simulink model "MCuC_Harness"  (R2025b)
settings: Solver=ode8  StartTime=0.0  StopTime=10.0  FixedStep=.0001  RelTol=1e-3
undefined symbols (not defined in the file): BMS_Contactor_Command, MC_DC_State, MC_VSM_State, UC_State
libraries: simulink x5
settings Model: DataDictionary=rev3_data.sldd  Creator=matat  LastModifiedBy=matat
settings OptimizationCC: DefaultParameterBehavior=Inlined  EnhancedBackFolding=on  PassReuseOutputArgsThreshold=0.0  OptimizeBlockOrder=speed  DifferentSizesBufferReuse=on  OptimizationCustomize=off
settings DebuggingCC: ParameterTunabilityLossMsg=error
settings SFSimCC: MATLABDynamicMemAlloc=off
settings RTWCC: GPUComputeCapability=3.5
settings CodeAppCC: ForceParamTrailComments=on  OperatorAnnotations=on

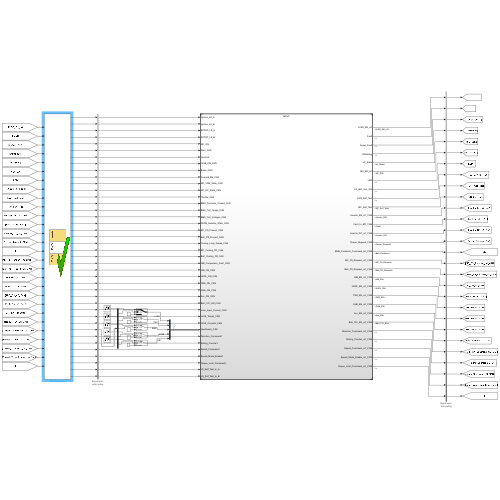
[thumbnail: Simulink's stored preview of the top-level diagram]
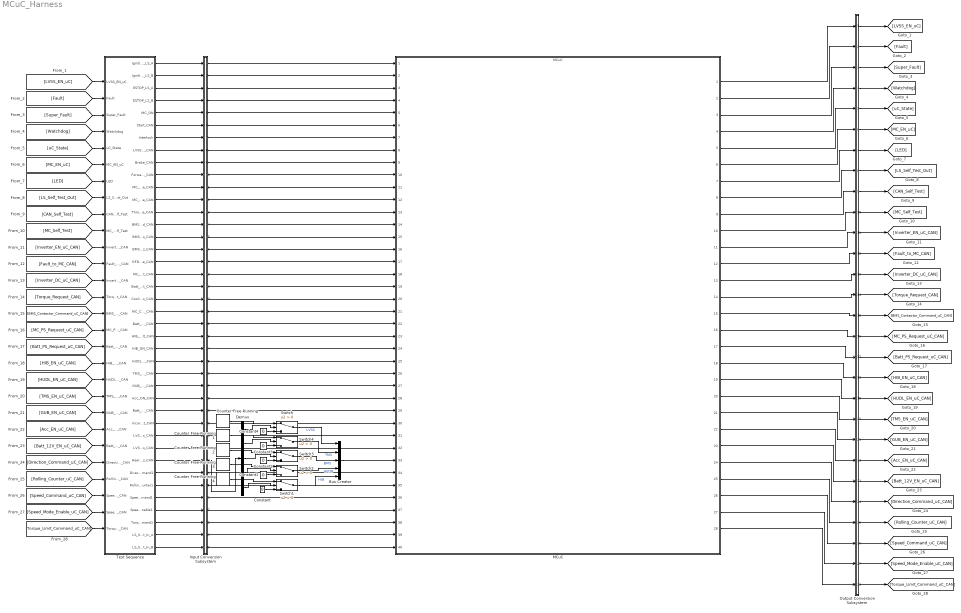
== system MCuC_Harness ==
  Bus Creator : BusCreator  Inputs=5
  Constant{,1..4} (5 alike) : Constant  Value=0
  Counter Free-Running{,1..4} (5 alike) : simulink/Sources/Counter Free-Running  NumBits=32  tsamp=-1
  Demux : Demux  Outputs=5
  Input Conversion Subsystem : Subsystem  Tag=__SLT_ICS__  Description=|
      | Signal spec.
      | and routing
      settings: AttributesFormatString=%<Description>
  MCuC : ModelReference  ModelNameDialog=MCuC  SimulationMode=Normal  ModelReferenceVersion=5.2
  Output Conversion Subsystem : Subsystem  Tag=__SLT_OCS__  Description=|
      | Signal spec.
      | and routing
      settings: AttributesFormatString=%<Description>
  Switch{,1..4} (5 alike) : Switch  Criteria=u2 > Threshold  SaturateOnIntegerOverflow=off  InputSameDT=off
  Test Sequence : Test Sequence  TreatAsAtomicUnit=on
  wires:
  Test Sequence/1(Ignition_LS_A) -> Input Conversion Subsystem/1(Inport_1)
  Test Sequence/2(Ignition_LS_B) -> Input Conversion Subsystem/2(Inport_2)
  Test Sequence/3(ESTOP_LS_A) -> Input Conversion Subsystem/3(Inport_3)
  Test Sequence/4(ESTOP_LS_B) -> Input Conversion Subsystem/4(Inport_4)
  Test Sequence/5(MC_ON) -> Input Conversion Subsystem/5(Inport_5)
  Test Sequence/6(Start_CAN) -> Input Conversion Subsystem/6(Inport_6)
  Test Sequence/7(Interlock) -> Input Conversion Subsystem/7(Inport_7)
  Test Sequence/8(LVSS_ON_CAN) -> Input Conversion Subsystem/8(Inport_8)
  Test Sequence/9(Brake_CAN) -> Input Conversion Subsystem/9(Inport_9)
  Test Sequence/10(Forward_EN_CAN) -> Input Conversion Subsystem/10(Inport_10)
  Test Sequence/11(MC_VSM_State_CAN) -> Input Conversion Subsystem/11(Inport_11)
  Test Sequence/12(MC_DC_State_CAN) -> Input Conversion Subsystem/12(Inport_12)
  Test Sequence/13(Throttle_CAN) -> Input Conversion Subsystem/13(Inport_13)
  Test Sequence/14(BMS_Contactor_Closed_CAN) -> Input Conversion Subsystem/14(Inport_14)
  Test Sequence/15(BMS_Cell_Temps_CAN) -> Input Conversion Subsystem/15(Inport_15)
  Test Sequence/16(BMS_Cell_Voltages_CAN) -> Input Conversion Subsystem/16(Inport_16)
  Test Sequence/17(GFDB_Isolation_State_CAN) -> Input Conversion Subsystem/17(Inport_17)
  Test Sequence/18(MC_PS_Present_CAN) -> Input Conversion Subsystem/18(Inport_18)
  Test Sequence/19(Batt_PS_Present_CAN) -> Input Conversion Subsystem/19(Inport_19)
  Test Sequence/20(Cooling_Loop_Temps_CAN) -> Input Conversion Subsystem/20(Inport_20)
  Test Sequence/21(MC_Cooling_FR_CAN) -> Input Conversion Subsystem/21(Inport_21)
  Test Sequence/22(Batt_Cooling_FR_CAN) -> Input Conversion Subsystem/22(Inport_22)
  Test Sequence/23(HIB_Comparison_Fault_CAN) -> Input Conversion Subsystem/23(Inport_23)
  Test Sequence/24(HIB_ON_CAN) -> Input Conversion Subsystem/24(Inport_24)
  Test Sequence/25(HUDL_ON_CAN) -> Input Conversion Subsystem/25(Inport_25)
  Test Sequence/26(TMS_ON_CAN) -> Input Conversion Subsystem/26(Inport_26)
  Test Sequence/27(GUB_ON_CAN) -> Input Conversion Subsystem/27(Inport_27)
  Test Sequence/28(Acc_ON_CAN) -> Input Conversion Subsystem/28(Inport_28)
  Test Sequence/29(Batt_12V_ON_CAN) -> Input Conversion Subsystem/29(Inport_29)
  Test Sequence/30(Vicor_Input_Current_CAN) -> Input Conversion Subsystem/30(Inport_30)
  Test Sequence/31(LVSS_Temps_CAN) -> Input Conversion Subsystem/31(Inport_31)
  Test Sequence/32(LVSS_Currents_CAN) -> Input Conversion Subsystem/32(Inport_32)
  Test Sequence/34(Direction_Command1) -> Input Conversion Subsystem/34(Inport_34)
  Test Sequence/35(Rolling_Counter1) -> Input Conversion Subsystem/35(Inport_35)
  Test Sequence/36(Speed_Command1) -> Input Conversion Subsystem/36(Inport_36)
  Test Sequence/37(Speed_Mode_Enable1) -> Input Conversion Subsystem/37(Inport_37)
  Test Sequence/38(Torque_Limit_Command1) -> Input Conversion Subsystem/38(Inport_38)
  Test Sequence/39(LS_Self_Test_In_A) -> Input Conversion Subsystem/39(Inport_39)
  Test Sequence/40(LS_Self_Test_In_B) -> Input Conversion Subsystem/40(Inport_40)
  [LVSS_EN_uC] -> Test Sequence/1(LVSS_EN_uC)
  [Fault] -> Test Sequence/2(Fault)
  [Super_Fault] -> Test Sequence/3(Super_Fault)
  [Watchdog] -> Test Sequence/4(Watchdog)
  [uC_State] -> Test Sequence/5(uC_State)
  [MC_EN_uC] -> Test Sequence/6(MC_EN_uC)
  [LED] -> Test Sequence/7(LED)
  [LS_Self_Test_Out] -> Test Sequence/8(LS_Self_Test_Out)
  [CAN_Self_Test] -> Test Sequence/9(CAN_Self_Test)
  [MC_Self_Test] -> Test Sequence/10(MC_Self_Test)
  [Inverter_EN_uC_CAN] -> Test Sequence/11(Inverter_EN_uC_CAN)
  [Fault_to_MC_CAN] -> Test Sequence/12(Fault_to_MC_CAN)
  [Inverter_DC_uC_CAN] -> Test Sequence/13(Inverter_DC_uC_CAN)
  [Torque_Request_CAN] -> Test Sequence/14(Torque_Request_CAN)
  [BMS_Contactor_Command_uC_CAN] -> Test Sequence/15(BMS_Contactor_Command_uC_CAN)
  [MC_PS_Request_uC_CAN] -> Test Sequence/16(MC_PS_Request_uC_CAN)
  [Batt_PS_Request_uC_CAN] -> Test Sequence/17(Batt_PS_Request_uC_CAN)
  [HIB_EN_uC_CAN] -> Test Sequence/18(HIB_EN_uC_CAN)
  [HUDL_EN_uC_CAN] -> Test Sequence/19(HUDL_EN_uC_CAN)
  [TMS_EN_uC_CAN] -> Test Sequence/20(TMS_EN_uC_CAN)
  [GUB_EN_uC_CAN] -> Test Sequence/21(GUB_EN_uC_CAN)
  [Acc_EN_uC_CAN] -> Test Sequence/22(Acc_EN_uC_CAN)
  [Batt_12V_EN_uC_CAN] -> Test Sequence/23(Batt_12V_EN_uC_CAN)
  [Direction_Command_uC_CAN] -> Test Sequence/24(Direction_Command_uC_CAN)
  [Rolling_Counter_uC_CAN] -> Test Sequence/25(Rolling_Counter_uC_CAN)
  [Speed_Command_uC_CAN] -> Test Sequence/26(Speed_Command_uC_CAN)
  [Speed_Mode_Enable_uC_CAN] -> Test Sequence/27(Speed_Mode_Enable_uC_CAN)
  [Torque_Limit_Command_uC_CAN] -> Test Sequence/28(Torque_Limit_Command_uC_CAN)
  Output Conversion Subsystem/1(Outport_1) -> [LVSS_EN_uC]
  Output Conversion Subsystem/2(Outport_2) -> [Fault]
  Output Conversion Subsystem/3(Outport_3) -> [Super_Fault]
  Output Conversion Subsystem/4(Outport_4) -> [Watchdog]
  Output Conversion Subsystem/5(Outport_5) -> [uC_State]
  Output Conversion Subsystem/6(Outport_6) -> [MC_EN_uC]
  Output Conversion Subsystem/7(Outport_7) -> [LED]
  Output Conversion Subsystem/8(Outport_8) -> [LS_Self_Test_Out]
  Output Conversion Subsystem/9(Outport_9) -> [CAN_Self_Test]
  Output Conversion Subsystem/10(Outport_10) -> [MC_Self_Test]
  Output Conversion Subsystem/11(Outport_11) -> [Inverter_EN_uC_CAN]
  Output Conversion Subsystem/12(Outport_12) -> [Fault_to_MC_CAN]
  Output Conversion Subsystem/13(Outport_13) -> [Inverter_DC_uC_CAN]
  Output Conversion Subsystem/14(Outport_14) -> [Torque_Request_CAN]
  Output Conversion Subsystem/15(Outport_15) -> [BMS_Contactor_Command_uC_CAN]
  Output Conversion Subsystem/16(Outport_16) -> [MC_PS_Request_uC_CAN]
  Output Conversion Subsystem/17(Outport_17) -> [Batt_PS_Request_uC_CAN]
  Output Conversion Subsystem/18(Outport_18) -> [HIB_EN_uC_CAN]
  Output Conversion Subsystem/19(Outport_19) -> [HUDL_EN_uC_CAN]
  Output Conversion Subsystem/20(Outport_20) -> [TMS_EN_uC_CAN]
  Output Conversion Subsystem/21(Outport_21) -> [GUB_EN_uC_CAN]
  Output Conversion Subsystem/22(Outport_22) -> [Acc_EN_uC_CAN]
  Output Conversion Subsystem/23(Outport_23) -> [Batt_12V_EN_uC_CAN]
  Output Conversion Subsystem/24(Outport_24) -> [Direction_Command_uC_CAN]
  Output Conversion Subsystem/25(Outport_25) -> [Rolling_Counter_uC_CAN]
  Output Conversion Subsystem/26(Outport_26) -> [Speed_Command_uC_CAN]
  Output Conversion Subsystem/27(Outport_27) -> [Speed_Mode_Enable_uC_CAN]
  Output Conversion Subsystem/28(Outport_28) -> [Torque_Limit_Command_uC_CAN]
  Input Conversion Subsystem/1(Outport_1) -> MCuC/1
  Input Conversion Subsystem/2(Outport_2) -> MCuC/2
  Input Conversion Subsystem/3(Outport_3) -> MCuC/3
  Input Conversion Subsystem/4(Outport_4) -> MCuC/4
  Input Conversion Subsystem/5(Outport_5) -> MCuC/5
  Input Conversion Subsystem/6(Outport_6) -> MCuC/6
  Input Conversion Subsystem/7(Outport_7) -> MCuC/7
  Input Conversion Subsystem/8(Outport_8) -> MCuC/8
  Input Conversion Subsystem/9(Outport_9) -> MCuC/9
  Input Conversion Subsystem/10(Outport_10) -> MCuC/10
  Input Conversion Subsystem/11(Outport_11) -> MCuC/11
  Input Conversion Subsystem/12(Outport_12) -> MCuC/12
  Input Conversion Subsystem/13(Outport_13) -> MCuC/13
  Input Conversion Subsystem/14(Outport_14) -> MCuC/14
  Input Conversion Subsystem/15(Outport_15) -> MCuC/15
  Input Conversion Subsystem/16(Outport_16) -> MCuC/16
  Input Conversion Subsystem/17(Outport_17) -> MCuC/17
  Input Conversion Subsystem/18(Outport_18) -> MCuC/18
  Input Conversion Subsystem/19(Outport_19) -> MCuC/19
  Input Conversion Subsystem/20(Outport_20) -> MCuC/20
  Input Conversion Subsystem/21(Outport_21) -> MCuC/21
  Input Conversion Subsystem/22(Outport_22) -> MCuC/22
  Input Conversion Subsystem/23(Outport_23) -> MCuC/23
  Input Conversion Subsystem/24(Outport_24) -> MCuC/24
  Input Conversion Subsystem/25(Outport_25) -> MCuC/25
  Input Conversion Subsystem/26(Outport_26) -> MCuC/26
  Input Conversion Subsystem/27(Outport_27) -> MCuC/27
  Input Conversion Subsystem/28(Outport_28) -> MCuC/28
  Input Conversion Subsystem/29(Outport_29) -> MCuC/29
  Input Conversion Subsystem/30(Outport_30) -> MCuC/30
  Input Conversion Subsystem/31(Outport_31) -> MCuC/31
  Input Conversion Subsystem/32(Outport_32) -> MCuC/32
  Input Conversion Subsystem/34(Outport_34) -> MCuC/34
  Input Conversion Subsystem/35(Outport_35) -> MCuC/35
  Input Conversion Subsystem/36(Outport_36) -> MCuC/36
  Input Conversion Subsystem/37(Outport_37) -> MCuC/37
  Input Conversion Subsystem/38(Outport_38) -> MCuC/38
  Input Conversion Subsystem/39(Outport_39) -> MCuC/39
  Input Conversion Subsystem/40(Outport_40) -> MCuC/40
  MCuC/1 -> Output Conversion Subsystem/1(Inport_1)
  MCuC/2 -> Output Conversion Subsystem/2(Inport_2)
  MCuC/3 -> Output Conversion Subsystem/3(Inport_3)
  MCuC/4 -> Output Conversion Subsystem/4(Inport_4)
  MCuC/5 -> Output Conversion Subsystem/5(Inport_5)
  MCuC/6 -> Output Conversion Subsystem/6(Inport_6)
  MCuC/7 -> Output Conversion Subsystem/7(Inport_7)
  MCuC/8 -> Output Conversion Subsystem/8(Inport_8)
  MCuC/9 -> Output Conversion Subsystem/9(Inport_9)
  MCuC/10 -> Output Conversion Subsystem/10(Inport_10)
  MCuC/11 -> Output Conversion Subsystem/11(Inport_11)
  MCuC/12 -> Output Conversion Subsystem/12(Inport_12)
  MCuC/13 -> Output Conversion Subsystem/13(Inport_13)
  MCuC/14 -> Output Conversion Subsystem/14(Inport_14)
  MCuC/15 -> Output Conversion Subsystem/15(Inport_15)
  MCuC/16 -> Output Conversion Subsystem/16(Inport_16)
  MCuC/17 -> Output Conversion Subsystem/17(Inport_17)
  MCuC/18 -> Output Conversion Subsystem/18(Inport_18)
  MCuC/19 -> Output Conversion Subsystem/19(Inport_19)
  MCuC/20 -> Output Conversion Subsystem/20(Inport_20)
  MCuC/21 -> Output Conversion Subsystem/21(Inport_21)
  MCuC/22 -> Output Conversion Subsystem/22(Inport_22)
  MCuC/23 -> Output Conversion Subsystem/23(Inport_23)
  MCuC/24 -> Output Conversion Subsystem/24(Inport_24)
  MCuC/25 -> Output Conversion Subsystem/25(Inport_25)
  MCuC/26 -> Output Conversion Subsystem/26(Inport_26)
  MCuC/27 -> Output Conversion Subsystem/27(Inport_27)
  MCuC/28 -> Output Conversion Subsystem/28(Inport_28)
  Counter Free-Running/1 -> Switch/1
  Counter Free-Running1/1 -> Switch4/1
  Counter Free-Running2/1 -> Switch3/1
  Counter Free-Running3/1 -> Switch2/1
  Counter Free-Running4/1 -> Switch1/1
  Constant/1 -> Switch1/3
  Constant4/1 -> Switch/3
  Constant3/1 -> Switch4/3
  Constant2/1 -> Switch3/3
  Constant1/1 -> Switch2/3
  Test Sequence/33(Heartbeats_CAN) -> Input Conversion Subsystem/33(Inport_33)
  Input Conversion Subsystem/33(Outport_33) -> Demux/1
  Demux/1 -> Switch/2
  Demux/2 -> Switch4/2
  Demux/3 -> Switch3/2
  Demux/4 -> Switch2/2
  Demux/5 -> Switch1/2
  Switch/1 -> Bus Creator/1  "LVSS"
  Switch4/1 -> Bus Creator/2  "TMS"
  Switch3/1 -> Bus Creator/3  "BMS"
  Switch2/1 -> Bus Creator/4  "GFDB"
  Switch1/1 -> Bus Creator/5  "HIB"
  Bus Creator/1 -> MCuC/33

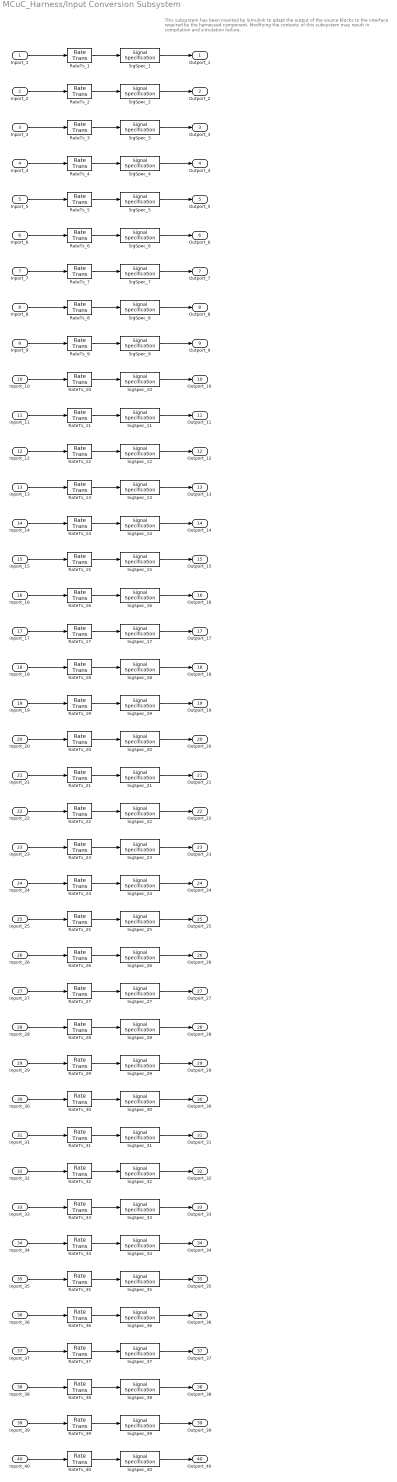
== system MCuC_Harness/Input Conversion Subsystem ==
  note: This subsystem has been inserted by Simulink to adapt the output of the source blocks to the interface required by the harnessed component.
      |  Modifying the contents of this subsystem may result in compilation and simulation failure.
  Inport_1 : Inport
  Inport_2 : Inport  Port=2
  Inport_3 : Inport  Port=3
  Inport_4 : Inport  Port=4
  Inport_5 : Inport  Port=5
  Inport_6 : Inport  Port=6
  Inport_7 : Inport  Port=7
  Inport_8 : Inport  Port=8
  Inport_9 : Inport  Port=9
  Inport_10 : Inport  Port=10
  Inport_11 : Inport  Port=11
  Inport_12 : Inport  Port=12
  Inport_13 : Inport  Port=13
  Inport_14 : Inport  Port=14
  Inport_15 : Inport  Port=15
  Inport_16 : Inport  Port=16
  Inport_17 : Inport  Port=17
  Inport_18 : Inport  Port=18
  Inport_19 : Inport  Port=19
  Inport_20 : Inport  Port=20
  Inport_21 : Inport  Port=21
  Inport_22 : Inport  Port=22
  Inport_23 : Inport  Port=23
  Inport_24 : Inport  Port=24
  Inport_25 : Inport  Port=25
  Inport_26 : Inport  Port=26
  Inport_27 : Inport  Port=27
  Inport_28 : Inport  Port=28
  Inport_29 : Inport  Port=29
  Inport_30 : Inport  Port=30
  Inport_31 : Inport  Port=31
  Inport_32 : Inport  Port=32
  Inport_33 : Inport  Port=33
  Inport_34 : Inport  Port=34
  Inport_35 : Inport  Port=35
  Inport_36 : Inport  Port=36
  Inport_37 : Inport  Port=37
  Inport_38 : Inport  Port=38
  Inport_39 : Inport  Port=39
  Inport_40 : Inport  Port=40
  RateTs_{1..10,13..40} (38 alike) : RateTransition  OutPortSampleTime=0.0001
  RateTs_11 : RateTransition  InitialCondition=MC_VSM_State.Start  OutPortSampleTime=0.0001
  RateTs_12 : RateTransition  InitialCondition=MC_DC_State.Disabled  OutPortSampleTime=0.0001
  SigSpec_{1..10,14,23..29,39..40} (20 alike) : SignalSpecification  OutDataTypeStr=boolean  Dimensions=[1]  SampleTime=0.0001
  SigSpec_11 : SignalSpecification  OutDataTypeStr=Enum: MC_VSM_State  Dimensions=[1]  SampleTime=0.0001
  SigSpec_12 : SignalSpecification  OutDataTypeStr=Enum: MC_DC_State  Dimensions=[1]  SampleTime=0.0001
  SigSpec_{13,21..22,30,34..38} (9 alike) : SignalSpecification  OutDataTypeStr=int16  Dimensions=[1]  SampleTime=0.0001
  SigSpec_15 : SignalSpecification  OutDataTypeStr=int32  Dimensions=[1, 45]  SampleTime=0.0001
  SigSpec_16 : SignalSpecification  OutDataTypeStr=int16  Dimensions=[1, 100]  SampleTime=0.0001
  SigSpec_17 : SignalSpecification  OutDataTypeStr=uint8  Dimensions=[1]  SampleTime=0.0001
  SigSpec_18 : SignalSpecification  OutDataTypeStr=uint8  Dimensions=[1]  SampleTime=0.0001
  SigSpec_19 : SignalSpecification  OutDataTypeStr=uint8  Dimensions=[1]  SampleTime=0.0001
  SigSpec_20 : SignalSpecification  OutDataTypeStr=int32  Dimensions=[1, 5]  SampleTime=0.0001
  SigSpec_31 : SignalSpecification  OutDataTypeStr=int32  Dimensions=[1, 6]  SampleTime=0.0001
  SigSpec_32 : SignalSpecification  OutDataTypeStr=int16  Dimensions=[1, 6]  SampleTime=0.0001
  SigSpec_33 : SignalSpecification  OutDataTypeStr=uint32  Dimensions=[1, 5]  SampleTime=0.0001
  Outport_1 : Outport
  Outport_2 : Outport  Port=2
  Outport_3 : Outport  Port=3
  Outport_4 : Outport  Port=4
  Outport_5 : Outport  Port=5
  Outport_6 : Outport  Port=6
  Outport_7 : Outport  Port=7
  Outport_8 : Outport  Port=8
  Outport_9 : Outport  Port=9
  Outport_10 : Outport  Port=10
  Outport_11 : Outport  Port=11
  Outport_12 : Outport  Port=12
  Outport_13 : Outport  Port=13
  Outport_14 : Outport  Port=14
  Outport_15 : Outport  Port=15
  Outport_16 : Outport  Port=16
  Outport_17 : Outport  Port=17
  Outport_18 : Outport  Port=18
  Outport_19 : Outport  Port=19
  Outport_20 : Outport  Port=20
  Outport_21 : Outport  Port=21
  Outport_22 : Outport  Port=22
  Outport_23 : Outport  Port=23
  Outport_24 : Outport  Port=24
  Outport_25 : Outport  Port=25
  Outport_26 : Outport  Port=26
  Outport_27 : Outport  Port=27
  Outport_28 : Outport  Port=28
  Outport_29 : Outport  Port=29
  Outport_30 : Outport  Port=30
  Outport_31 : Outport  Port=31
  Outport_32 : Outport  Port=32
  Outport_33 : Outport  Port=33
  Outport_34 : Outport  Port=34
  Outport_35 : Outport  Port=35
  Outport_36 : Outport  Port=36
  Outport_37 : Outport  Port=37
  Outport_38 : Outport  Port=38
  Outport_39 : Outport  Port=39
  Outport_40 : Outport  Port=40
  wires:
  SigSpec_1/1 -> Outport_1/1
  RateTs_1/1 -> SigSpec_1/1
  Inport_1/1 -> RateTs_1/1
  SigSpec_2/1 -> Outport_2/1
  RateTs_2/1 -> SigSpec_2/1
  Inport_2/1 -> RateTs_2/1
  SigSpec_3/1 -> Outport_3/1
  RateTs_3/1 -> SigSpec_3/1
  Inport_3/1 -> RateTs_3/1
  SigSpec_4/1 -> Outport_4/1
  RateTs_4/1 -> SigSpec_4/1
  Inport_4/1 -> RateTs_4/1
  SigSpec_5/1 -> Outport_5/1
  RateTs_5/1 -> SigSpec_5/1
  Inport_5/1 -> RateTs_5/1
  SigSpec_6/1 -> Outport_6/1
  RateTs_6/1 -> SigSpec_6/1
  Inport_6/1 -> RateTs_6/1
  SigSpec_7/1 -> Outport_7/1
  RateTs_7/1 -> SigSpec_7/1
  Inport_7/1 -> RateTs_7/1
  SigSpec_8/1 -> Outport_8/1
  RateTs_8/1 -> SigSpec_8/1
  Inport_8/1 -> RateTs_8/1
  SigSpec_9/1 -> Outport_9/1
  RateTs_9/1 -> SigSpec_9/1
  Inport_9/1 -> RateTs_9/1
  SigSpec_10/1 -> Outport_10/1
  RateTs_10/1 -> SigSpec_10/1
  Inport_10/1 -> RateTs_10/1
  SigSpec_11/1 -> Outport_11/1
  RateTs_11/1 -> SigSpec_11/1
  Inport_11/1 -> RateTs_11/1
  SigSpec_12/1 -> Outport_12/1
  RateTs_12/1 -> SigSpec_12/1
  Inport_12/1 -> RateTs_12/1
  SigSpec_13/1 -> Outport_13/1
  RateTs_13/1 -> SigSpec_13/1
  Inport_13/1 -> RateTs_13/1
  SigSpec_14/1 -> Outport_14/1
  RateTs_14/1 -> SigSpec_14/1
  Inport_14/1 -> RateTs_14/1
  SigSpec_15/1 -> Outport_15/1
  RateTs_15/1 -> SigSpec_15/1
  Inport_15/1 -> RateTs_15/1
  SigSpec_16/1 -> Outport_16/1
  RateTs_16/1 -> SigSpec_16/1
  Inport_16/1 -> RateTs_16/1
  SigSpec_17/1 -> Outport_17/1
  RateTs_17/1 -> SigSpec_17/1
  Inport_17/1 -> RateTs_17/1
  SigSpec_18/1 -> Outport_18/1
  RateTs_18/1 -> SigSpec_18/1
  Inport_18/1 -> RateTs_18/1
  SigSpec_19/1 -> Outport_19/1
  RateTs_19/1 -> SigSpec_19/1
  Inport_19/1 -> RateTs_19/1
  SigSpec_20/1 -> Outport_20/1
  RateTs_20/1 -> SigSpec_20/1
  Inport_20/1 -> RateTs_20/1
  SigSpec_21/1 -> Outport_21/1
  RateTs_21/1 -> SigSpec_21/1
  Inport_21/1 -> RateTs_21/1
  SigSpec_22/1 -> Outport_22/1
  RateTs_22/1 -> SigSpec_22/1
  Inport_22/1 -> RateTs_22/1
  SigSpec_23/1 -> Outport_23/1
  RateTs_23/1 -> SigSpec_23/1
  Inport_23/1 -> RateTs_23/1
  SigSpec_24/1 -> Outport_24/1
  RateTs_24/1 -> SigSpec_24/1
  Inport_24/1 -> RateTs_24/1
  SigSpec_25/1 -> Outport_25/1
  RateTs_25/1 -> SigSpec_25/1
  Inport_25/1 -> RateTs_25/1
  SigSpec_26/1 -> Outport_26/1
  RateTs_26/1 -> SigSpec_26/1
  Inport_26/1 -> RateTs_26/1
  SigSpec_27/1 -> Outport_27/1
  RateTs_27/1 -> SigSpec_27/1
  Inport_27/1 -> RateTs_27/1
  SigSpec_28/1 -> Outport_28/1
  RateTs_28/1 -> SigSpec_28/1
  Inport_28/1 -> RateTs_28/1
  SigSpec_29/1 -> Outport_29/1
  RateTs_29/1 -> SigSpec_29/1
  Inport_29/1 -> RateTs_29/1
  SigSpec_30/1 -> Outport_30/1
  RateTs_30/1 -> SigSpec_30/1
  Inport_30/1 -> RateTs_30/1
  SigSpec_31/1 -> Outport_31/1
  RateTs_31/1 -> SigSpec_31/1
  Inport_31/1 -> RateTs_31/1
  SigSpec_32/1 -> Outport_32/1
  RateTs_32/1 -> SigSpec_32/1
  Inport_32/1 -> RateTs_32/1
  SigSpec_33/1 -> Outport_33/1
  RateTs_33/1 -> SigSpec_33/1
  Inport_33/1 -> RateTs_33/1
  SigSpec_34/1 -> Outport_34/1
  RateTs_34/1 -> SigSpec_34/1
  Inport_34/1 -> RateTs_34/1
  SigSpec_35/1 -> Outport_35/1
  RateTs_35/1 -> SigSpec_35/1
  Inport_35/1 -> RateTs_35/1
  SigSpec_36/1 -> Outport_36/1
  RateTs_36/1 -> SigSpec_36/1
  Inport_36/1 -> RateTs_36/1
  SigSpec_37/1 -> Outport_37/1
  RateTs_37/1 -> SigSpec_37/1
  Inport_37/1 -> RateTs_37/1
  SigSpec_38/1 -> Outport_38/1
  RateTs_38/1 -> SigSpec_38/1
  Inport_38/1 -> RateTs_38/1
  SigSpec_39/1 -> Outport_39/1
  RateTs_39/1 -> SigSpec_39/1
  Inport_39/1 -> RateTs_39/1
  SigSpec_40/1 -> Outport_40/1
  RateTs_40/1 -> SigSpec_40/1
  Inport_40/1 -> RateTs_40/1

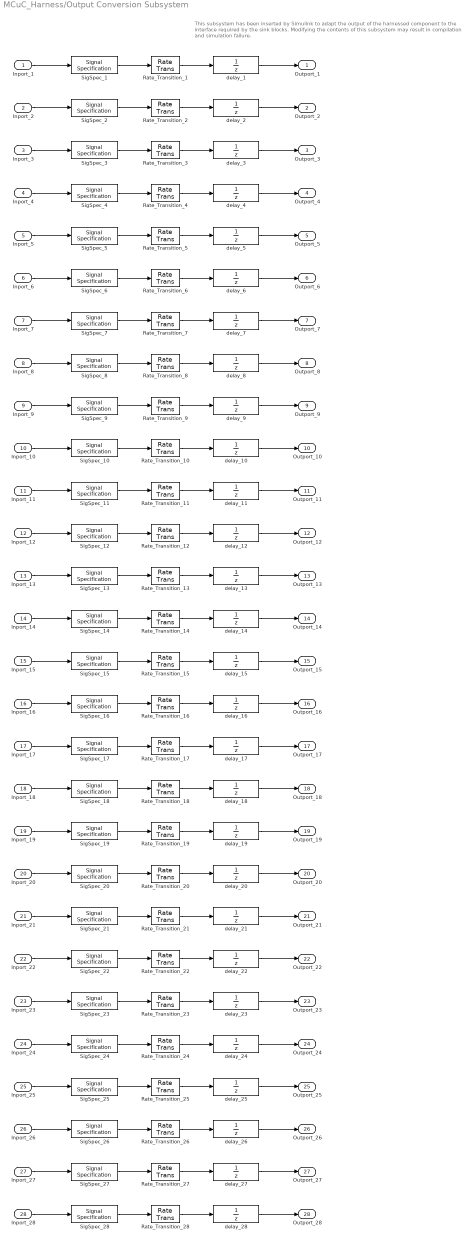
== system MCuC_Harness/Output Conversion Subsystem ==
  note: This subsystem has been inserted by Simulink to adapt the output of the harnessed component to the interface required by the sink blocks.
      |  Modifying the contents of this subsystem may result in compilation and simulation failure.
  Inport_1 : Inport
  Inport_2 : Inport  Port=2
  Inport_3 : Inport  Port=3
  Inport_4 : Inport  Port=4
  Inport_5 : Inport  Port=5
  Inport_6 : Inport  Port=6
  Inport_7 : Inport  Port=7
  Inport_8 : Inport  Port=8
  Inport_9 : Inport  Port=9
  Inport_10 : Inport  Port=10
  Inport_11 : Inport  Port=11
  Inport_12 : Inport  Port=12
  Inport_13 : Inport  Port=13
  Inport_14 : Inport  Port=14
  Inport_15 : Inport  Port=15
  Inport_16 : Inport  Port=16
  Inport_17 : Inport  Port=17
  Inport_18 : Inport  Port=18
  Inport_19 : Inport  Port=19
  Inport_20 : Inport  Port=20
  Inport_21 : Inport  Port=21
  Inport_22 : Inport  Port=22
  Inport_23 : Inport  Port=23
  Inport_24 : Inport  Port=24
  Inport_25 : Inport  Port=25
  Inport_26 : Inport  Port=26
  Inport_27 : Inport  Port=27
  Inport_28 : Inport  Port=28
  Rate_Transition_{1..4,6..14,16..28} (26 alike) : RateTransition  OutPortSampleTimeOpt=Inherit
  Rate_Transition_15 : RateTransition  InitialCondition=BMS_Contactor_Command.Open_Contactor  OutPortSampleTimeOpt=Inherit
  Rate_Transition_5 : RateTransition  InitialCondition=UC_State.Preset  OutPortSampleTimeOpt=Inherit
  SigSpec_{1,4,6,11..13,18..23} (12 alike) : SignalSpecification  OutDataTypeStr=boolean  Dimensions=[1]  SampleTime=0.0001
  SigSpec_{2..3,8..10} (5 alike) : SignalSpecification  OutDataTypeStr=boolean  Dimensions=[1]
  SigSpec_{14,24..28} (6 alike) : SignalSpecification  OutDataTypeStr=int16  Dimensions=[1]  SampleTime=0.0001
  SigSpec_15 : SignalSpecification  OutDataTypeStr=Enum: BMS_Contactor_Command  Dimensions=[1]  SampleTime=0.0001
  SigSpec_16 : SignalSpecification  OutDataTypeStr=uint8  Dimensions=[1]  SampleTime=0.0001
  SigSpec_17 : SignalSpecification  OutDataTypeStr=uint8  Dimensions=[1]  SampleTime=0.0001
  SigSpec_5 : SignalSpecification  OutDataTypeStr=Enum: UC_State  Dimensions=[1]  SampleTime=0.0001
  SigSpec_7 : SignalSpecification  OutDataTypeStr=boolean  Dimensions=[1, 3]  SampleTime=0.0001
  delay_{1..4,6..14,16..28} (26 alike) : UnitDelay  SampleTime=-1
  delay_15 : UnitDelay  InitialCondition=BMS_Contactor_Command.Open_Contactor  SampleTime=-1
  delay_5 : UnitDelay  InitialCondition=UC_State.Preset  SampleTime=-1
  Outport_1 : Outport
  Outport_2 : Outport  Port=2
  Outport_3 : Outport  Port=3
  Outport_4 : Outport  Port=4
  Outport_5 : Outport  Port=5
  Outport_6 : Outport  Port=6
  Outport_7 : Outport  Port=7
  Outport_8 : Outport  Port=8
  Outport_9 : Outport  Port=9
  Outport_10 : Outport  Port=10
  Outport_11 : Outport  Port=11
  Outport_12 : Outport  Port=12
  Outport_13 : Outport  Port=13
  Outport_14 : Outport  Port=14
  Outport_15 : Outport  Port=15
  Outport_16 : Outport  Port=16
  Outport_17 : Outport  Port=17
  Outport_18 : Outport  Port=18
  Outport_19 : Outport  Port=19
  Outport_20 : Outport  Port=20
  Outport_21 : Outport  Port=21
  Outport_22 : Outport  Port=22
  Outport_23 : Outport  Port=23
  Outport_24 : Outport  Port=24
  Outport_25 : Outport  Port=25
  Outport_26 : Outport  Port=26
  Outport_27 : Outport  Port=27
  Outport_28 : Outport  Port=28
  wires:
  Inport_1/1 -> SigSpec_1/1
  SigSpec_1/1 -> Rate_Transition_1/1
  Rate_Transition_1/1 -> delay_1/1
  delay_1/1 -> Outport_1/1
  Inport_2/1 -> SigSpec_2/1
  SigSpec_2/1 -> Rate_Transition_2/1
  Rate_Transition_2/1 -> delay_2/1
  delay_2/1 -> Outport_2/1
  Inport_3/1 -> SigSpec_3/1
  SigSpec_3/1 -> Rate_Transition_3/1
  Rate_Transition_3/1 -> delay_3/1
  delay_3/1 -> Outport_3/1
  Inport_4/1 -> SigSpec_4/1
  SigSpec_4/1 -> Rate_Transition_4/1
  Rate_Transition_4/1 -> delay_4/1
  delay_4/1 -> Outport_4/1
  Inport_5/1 -> SigSpec_5/1
  SigSpec_5/1 -> Rate_Transition_5/1
  Rate_Transition_5/1 -> delay_5/1
  delay_5/1 -> Outport_5/1
  Inport_6/1 -> SigSpec_6/1
  SigSpec_6/1 -> Rate_Transition_6/1
  Rate_Transition_6/1 -> delay_6/1
  delay_6/1 -> Outport_6/1
  Inport_7/1 -> SigSpec_7/1
  SigSpec_7/1 -> Rate_Transition_7/1
  Rate_Transition_7/1 -> delay_7/1
  delay_7/1 -> Outport_7/1
  Inport_8/1 -> SigSpec_8/1
  SigSpec_8/1 -> Rate_Transition_8/1
  Rate_Transition_8/1 -> delay_8/1
  delay_8/1 -> Outport_8/1
  Inport_9/1 -> SigSpec_9/1
  SigSpec_9/1 -> Rate_Transition_9/1
  Rate_Transition_9/1 -> delay_9/1
  delay_9/1 -> Outport_9/1
  Inport_10/1 -> SigSpec_10/1
  SigSpec_10/1 -> Rate_Transition_10/1
  Rate_Transition_10/1 -> delay_10/1
  delay_10/1 -> Outport_10/1
  Inport_11/1 -> SigSpec_11/1
  SigSpec_11/1 -> Rate_Transition_11/1
  Rate_Transition_11/1 -> delay_11/1
  delay_11/1 -> Outport_11/1
  Inport_12/1 -> SigSpec_12/1
  SigSpec_12/1 -> Rate_Transition_12/1
  Rate_Transition_12/1 -> delay_12/1
  delay_12/1 -> Outport_12/1
  Inport_13/1 -> SigSpec_13/1
  SigSpec_13/1 -> Rate_Transition_13/1
  Rate_Transition_13/1 -> delay_13/1
  delay_13/1 -> Outport_13/1
  Inport_14/1 -> SigSpec_14/1
  SigSpec_14/1 -> Rate_Transition_14/1
  Rate_Transition_14/1 -> delay_14/1
  delay_14/1 -> Outport_14/1
  Inport_15/1 -> SigSpec_15/1
  SigSpec_15/1 -> Rate_Transition_15/1
  Rate_Transition_15/1 -> delay_15/1
  delay_15/1 -> Outport_15/1
  Inport_16/1 -> SigSpec_16/1
  SigSpec_16/1 -> Rate_Transition_16/1
  Rate_Transition_16/1 -> delay_16/1
  delay_16/1 -> Outport_16/1
  Inport_17/1 -> SigSpec_17/1
  SigSpec_17/1 -> Rate_Transition_17/1
  Rate_Transition_17/1 -> delay_17/1
  delay_17/1 -> Outport_17/1
  Inport_18/1 -> SigSpec_18/1
  SigSpec_18/1 -> Rate_Transition_18/1
  Rate_Transition_18/1 -> delay_18/1
  delay_18/1 -> Outport_18/1
  Inport_19/1 -> SigSpec_19/1
  SigSpec_19/1 -> Rate_Transition_19/1
  Rate_Transition_19/1 -> delay_19/1
  delay_19/1 -> Outport_19/1
  Inport_20/1 -> SigSpec_20/1
  SigSpec_20/1 -> Rate_Transition_20/1
  Rate_Transition_20/1 -> delay_20/1
  delay_20/1 -> Outport_20/1
  Inport_21/1 -> SigSpec_21/1
  SigSpec_21/1 -> Rate_Transition_21/1
  Rate_Transition_21/1 -> delay_21/1
  delay_21/1 -> Outport_21/1
  Inport_22/1 -> SigSpec_22/1
  SigSpec_22/1 -> Rate_Transition_22/1
  Rate_Transition_22/1 -> delay_22/1
  delay_22/1 -> Outport_22/1
  Inport_23/1 -> SigSpec_23/1
  SigSpec_23/1 -> Rate_Transition_23/1
  Rate_Transition_23/1 -> delay_23/1
  delay_23/1 -> Outport_23/1
  Inport_24/1 -> SigSpec_24/1
  SigSpec_24/1 -> Rate_Transition_24/1
  Rate_Transition_24/1 -> delay_24/1
  delay_24/1 -> Outport_24/1
  Inport_25/1 -> SigSpec_25/1
  SigSpec_25/1 -> Rate_Transition_25/1
  Rate_Transition_25/1 -> delay_25/1
  delay_25/1 -> Outport_25/1
  Inport_26/1 -> SigSpec_26/1
  SigSpec_26/1 -> Rate_Transition_26/1
  Rate_Transition_26/1 -> delay_26/1
  delay_26/1 -> Outport_26/1
  Inport_27/1 -> SigSpec_27/1
  SigSpec_27/1 -> Rate_Transition_27/1
  Rate_Transition_27/1 -> delay_27/1
  delay_27/1 -> Outport_27/1
  Inport_28/1 -> SigSpec_28/1
  SigSpec_28/1 -> Rate_Transition_28/1
  Rate_Transition_28/1 -> delay_28/1
  delay_28/1 -> Outport_28/1

== stateflow chart MCuC_Harness/Test Sequence ==
  state Basic_Operation_Cycle
    state Run
      %% Initialize data outputs.
      Ignition_LS_A = false;
      Ignition_LS_B = false;
      ESTOP_LS_A = false;
      ESTOP_LS_B = false;
      MC_ON = true;
      Start_CAN = false;
      Interlock = true;
      LVSS_ON_CAN = false;
      Brake_CAN = false;
      Forward_EN_CAN = false;
      MC_VSM_State_CAN = MC_VSM_State.Start;
      MC_DC_State_CAN = MC_DC_State.Disabled;
      Throttle_CAN = int16(0);
      BMS_Contactor_Closed_CAN = false;
      BMS_Cell_Temps_CAN = int32(zeros(1, 45));
      BMS_Cell_Voltages_CAN = int16(zeros(1, 100));
      GFDB_Isolation_State_CAN = uint8(0);
      MC_PS_Present_CAN = uint8(0);
      Batt_PS_Present_CAN = uint8(0);
      Cooling_Loop_Temps_CAN = int32(zeros(1, 5));
      MC_Cooling_FR_CAN = int16(0);
      Batt_Cooling_FR_CAN = int16(0);
      HIB_Comparison_Fault_CAN = false;
      HIB_ON_CAN = false;
      HUDL_ON_CAN = false;
      TMS_ON_CAN = false;
      GUB_ON_CAN = false;
      Acc_ON_CAN = false;
      Batt_12V_ON_CAN = false;
      Vicor_Input_Current_CAN = int16(0);
      LVSS_Temps_CAN = int32(zeros(1, 6));
      LVSS_Currents_CAN = int16(zeros(1, 6));
      Heartbeats_CAN = uint32([0, 0, 1, 1, 0]);
      Direction_Command1 = int16(0);
      Rolling_Counter1 = int16(0);
      Speed_Command1 = int16(0);
      Speed_Mode_Enable1 = int16(0);
      Torque_Limit_Command1 = int16(0);
      LS_Self_Test_In_A = false;
      LS_Self_Test_In_B = false;
      verify(BMS_Contactor_Command_uC_CAN == BMS_Contactor_Command.Open_Contactor);
    state Into_Key_Cycle
      BMS_Contactor_Closed_CAN = true;
      MC_ON = false;
    state MC_Off
      verify(LVSS_EN_uC == false);
      verify(Fault == false);
      verify(Super_Fault == false);
      verify(LS_Self_Test_Out == false);
      verify(CAN_Self_Test == false);
      verify(MC_Self_Test == false);
      verify(Inverter_EN_uC_CAN == false);
      verify(Fault_to_MC_CAN == false);
      verify(Inverter_DC_uC_CAN == false);
      verify(Torque_Request_CAN == 0);
      verify(BMS_Contactor_Command_uC_CAN == BMS_Contactor_Command.Close_Contactor);
      verify(MC_PS_Request_uC_CAN == false);
      verify(Batt_PS_Request_uC_CAN == false);
      verify(HIB_EN_uC_CAN == false);
      verify(HUDL_EN_uC_CAN == false);
      verify(TMS_EN_uC_CAN == false);
      verify(GUB_EN_uC_CAN == false);
      verify(Acc_EN_uC_CAN == false);
      verify(Batt_12V_EN_uC_CAN == false);
      verify(Direction_Command_uC_CAN == 0);
      verify(Rolling_Counter_uC_CAN == 0);
      verify(Speed_Command_uC_CAN == 0);
      verify(Speed_Mode_Enable_uC_CAN == 0);
      verify(Torque_Limit_Command_uC_CAN == 0);
      verify(MC_EN_uC == false);
      verify(all(LED ==  [false,true,false]))
      verify(uC_State == UC_State.MC_Off);
      verify(hasChanged(Watchdog) == true)
    state Transition_to_MC_Startup
      Ignition_LS_A = true;
      MC_ON = true;
    state LVSS_MC_Startup
      verify(LVSS_EN_uC == true);
      verify(MC_EN_uC == true);
      verify(uC_State == UC_State.LVSS_MC_Startup);
    state Transition_to_MC_Int
      LVSS_ON_CAN = true;
      Heartbeats_CAN = uint32([1, 0, 1, 1, 0]);
    state MC_Int
      verify(uC_State == UC_State.MC_Init);
      verify(TMS_EN_uC_CAN == true);
      verify(HUDL_EN_uC_CAN == true);
      verify(HIB_EN_uC_CAN == true);
      verify(Batt_12V_EN_uC_CAN == true);
      verify(GUB_EN_uC_CAN == true);
      verify(Acc_EN_uC_CAN == true);
    state Transition_to_Contactor_Closed
      MC_VSM_State_CAN = MC_VSM_State.Ready;
    state Contactor_Closed
      verify(Inverter_EN_uC_CAN == false);
      verify(uC_State == UC_State.Contactor_Closed);
    state Transition_to_MC_Ready
      Heartbeats_CAN = uint32([1, 1, 1, 1, 1]);
      Start_CAN = true;
    state MC_Ready
      verify(Inverter_EN_uC_CAN == false);
      verify(uC_State == UC_State.MC_Ready);
    state Transition_to_MC_Active
      Brake_CAN = true;
      Forward_EN_CAN = true;
      Throttle_CAN = 0;
    state MC_Active
      verify(all(LED ==  [true,false,false]))
      verify(uC_State == UC_State.MC_Active);
    state Transition_to_Contactor_Open
      Ignition_LS_A = false;
      Heartbeats_CAN = uint32([1, 0, 1, 1, 0]);
    state Contactor_Open
      verify(uC_State == UC_State.Contactor_Open);
      verify(TMS_EN_uC_CAN == false);
      verify(HUDL_EN_uC_CAN == false);
      verify(HIB_EN_uC_CAN == false);
      verify(Batt_12V_EN_uC_CAN == false);
      verify(GUB_EN_uC_CAN == false);
      verify(Acc_EN_uC_CAN == false);
      verify(Inverter_DC_uC_CAN == true);
      verify(Inverter_EN_uC_CAN == false);
    state Transition_to_MC_Discharge
      MC_DC_State_CAN = MC_DC_State.Disabled;
      MC_VSM_State_CAN = MC_VSM_State.Shutdown;
    state MC_Discharge
      verify(uC_State == UC_State.MC_Discharging);
    state Transition_to_LVSS_MC_Shutdown
      MC_DC_State_CAN = MC_DC_State.Complete;
      Heartbeats_CAN = uint32([0, 0, 1, 1, 0]);
    state LVSS_MC_Shutdown
      verify(uC_State == UC_State.LVSS_MC_Shutdown);
      verify(MC_EN_uC == false);
      verify(Inverter_DC_uC_CAN == false)
    (default) -> Run
    Run -> Basic_Operation_Cycle.Into_Key_Cycle : [
        | uC_State ~= UC_State.Preset
        | ]
    Basic_Operation_Cycle.Into_Key_Cycle -> MC_Off : [
        | uC_State ~= UC_State.Key_Cycle
        | ]
    MC_Off -> Transition_to_MC_Startup : [
        | after(1, sec)
        | ]
    Transition_to_MC_Startup -> LVSS_MC_Startup : [
        | after(1, sec)
        | ]
    LVSS_MC_Startup -> Transition_to_MC_Int : [
        | after(1, sec)
        | ]
    Transition_to_MC_Int -> MC_Int : [
        | after(1, sec)
        | ]
    MC_Int -> Transition_to_Contactor_Closed : [
        | after(1, sec)
        | ]
    Transition_to_Contactor_Closed -> Contactor_Closed : [
        | after(1, sec)
        | ]
    Contactor_Closed -> Transition_to_MC_Ready : [
        | after(1, sec)
        | ]
    Transition_to_MC_Ready -> MC_Ready : [
        | after(1, sec)
        | ]
    MC_Ready -> Transition_to_MC_Active : [
        | after(1, sec)
        | ]
    Transition_to_MC_Active -> MC_Active : [
        | after(1, sec)
        | ]
    MC_Active -> Transition_to_Contactor_Open : [
        | after(1, sec)
        | ]
    Transition_to_Contactor_Open -> Contactor_Open : [
        | after(1, sec)
        | ]
    Contactor_Open -> Transition_to_MC_Discharge : [
        | after(1, sec)
        | ]
    Transition_to_MC_Discharge -> MC_Discharge : [
        | after(1, sec)
        | ]
    MC_Discharge -> Transition_to_LVSS_MC_Shutdown : [
        | after(1, sec)
        | ]
    Transition_to_LVSS_MC_Shutdown -> LVSS_MC_Shutdown : [
        | after(1, sec)
        | ]
  state Heartbeat_Fault
    state Initialize
      Ignition_LS_A = false;
      Ignition_LS_B = false;
      ESTOP_LS_A = false;
      ESTOP_LS_B = false;
      MC_ON = true;
      Start_CAN = false;
      Interlock = true;
      LVSS_ON_CAN = false;
      Brake_CAN = false;
      Forward_EN_CAN = false;
      MC_VSM_State_CAN = MC_VSM_State.Start;
      MC_DC_State_CAN = MC_DC_State.Disabled;
      Throttle_CAN = int16(0);
      BMS_Contactor_Closed_CAN = false;
      BMS_Cell_Temps_CAN = int32(zeros(1, 45));
      BMS_Cell_Voltages_CAN = int16(zeros(1, 100));
      GFDB_Isolation_State_CAN = uint8(0);
      MC_PS_Present_CAN = uint8(0);
      Batt_PS_Present_CAN = uint8(0);
      Cooling_Loop_Temps_CAN = int32(zeros(1, 5));
      MC_Cooling_FR_CAN = int16(0);
      Batt_Cooling_FR_CAN = int16(0);
      HIB_Comparison_Fault_CAN = false;
      HIB_ON_CAN = false;
      HUDL_ON_CAN = false;
      TMS_ON_CAN = false;
      GUB_ON_CAN = false;
      Acc_ON_CAN = false;
      Batt_12V_ON_CAN = false;
      Vicor_Input_Current_CAN = int16(0);
      LVSS_Temps_CAN = int32(zeros(1, 6));
      LVSS_Currents_CAN = int16(zeros(1, 6));
      Heartbeats_CAN = uint32([0, 0, 1, 1, 0]);
      Direction_Command1 = int16(0);
      Rolling_Counter1 = int16(0);
      Speed_Command1 = int16(0);
      Speed_Mode_Enable1 = int16(0);
      Torque_Limit_Command1 = int16(0);
      LS_Self_Test_In_A = false;
      LS_Self_Test_In_B = false;
      verify(BMS_Contactor_Command_uC_CAN == BMS_Contactor_Command.Open_Contactor);
    state Into_Key_Cycle
      BMS_Contactor_Closed_CAN = true;
      MC_ON = false;
    state TMS
      TMS_ON_CAN = true;
      LVSS_ON_CAN = true;
      Heartbeats_CAN = uint32([1, 0, 1, 1, 0]);
    state Check
      verify(uC_State == UC_State.Fault);
    state Reset
      TMS_ON_CAN = false;
    state Check1
      verify(uC_State == UC_State.MC_Off);
    (default) -> Heartbeat_Fault.Initialize
    Heartbeat_Fault.Initialize -> Heartbeat_Fault.Into_Key_Cycle : [
        | uC_State ~= UC_State.Preset
        | ]
    Heartbeat_Fault.Into_Key_Cycle -> TMS : [
        | uC_State ~= UC_State.Key_Cycle
        | ]
    TMS -> Heartbeat_Fault.Check : [
        | after(1, sec)
        | ]
    Heartbeat_Fault.Check -> Reset : [
        | after(1, sec)
        | ]
    Reset -> Check1 : [
        | after(1, sec)
        | ]
  state MC_EN_Fault
    state Initialize
      Ignition_LS_A = false;
      Ignition_LS_B = false;
      ESTOP_LS_A = false;
      ESTOP_LS_B = false;
      MC_ON = true;
      Start_CAN = false;
      Interlock = true;
      LVSS_ON_CAN = false;
      Brake_CAN = false;
      Forward_EN_CAN = false;
      MC_VSM_State_CAN = MC_VSM_State.Start;
      MC_DC_State_CAN = MC_DC_State.Disabled;
      Throttle_CAN = int16(0);
      BMS_Contactor_Closed_CAN = false;
      BMS_Cell_Temps_CAN = int32(zeros(1, 45));
      BMS_Cell_Voltages_CAN = int16(zeros(1, 100));
      GFDB_Isolation_State_CAN = uint8(0);
      MC_PS_Present_CAN = uint8(0);
      Batt_PS_Present_CAN = uint8(0);
      Cooling_Loop_Temps_CAN = int32(zeros(1, 5));
      MC_Cooling_FR_CAN = int16(0);
      Batt_Cooling_FR_CAN = int16(0);
      HIB_Comparison_Fault_CAN = false;
      HIB_ON_CAN = false;
      HUDL_ON_CAN = false;
      TMS_ON_CAN = false;
      GUB_ON_CAN = false;
      Acc_ON_CAN = false;
      Batt_12V_ON_CAN = false;
      Vicor_Input_Current_CAN = int16(0);
      LVSS_Temps_CAN = int32(zeros(1, 6));
      LVSS_Currents_CAN = int16(zeros(1, 6));
      Heartbeats_CAN = uint32([0, 0, 1, 1, 0]);
      Direction_Command1 = int16(0);
      Rolling_Counter1 = int16(0);
      Speed_Command1 = int16(0);
      Speed_Mode_Enable1 = int16(0);
      Torque_Limit_Command1 = int16(0);
      LS_Self_Test_In_A = false;
      LS_Self_Test_In_B = false;
      verify(BMS_Contactor_Command_uC_CAN == BMS_Contactor_Command.Open_Contactor);
    state Into_Key_Cycle
      BMS_Contactor_Closed_CAN = true;
      MC_ON = false;
    state MC_Incorrect
      MC_ON = true;
    state Check
      verify(uC_State == UC_State.Fault);
    (default) -> MC_EN_Fault.Initialize
    MC_EN_Fault.Initialize -> MC_EN_Fault.Into_Key_Cycle : [
        | uC_State ~= UC_State.Preset
        | ]
    MC_EN_Fault.Into_Key_Cycle -> MC_EN_Fault.MC_Incorrect : [
        | uC_State ~= UC_State.Key_Cycle
        | ]
    MC_EN_Fault.MC_Incorrect -> MC_EN_Fault.Check : [
        | after(1, sec)
        | ]
  state GFDB_Fault
    state Initialize
      Ignition_LS_A = false;
      Ignition_LS_B = false;
      ESTOP_LS_A = false;
      ESTOP_LS_B = false;
      MC_ON = true;
      Start_CAN = false;
      Interlock = true;
      LVSS_ON_CAN = false;
      Brake_CAN = false;
      Forward_EN_CAN = false;
      MC_VSM_State_CAN = MC_VSM_State.Start;
      MC_DC_State_CAN = MC_DC_State.Disabled;
      Throttle_CAN = int16(0);
      BMS_Contactor_Closed_CAN = false;
      BMS_Cell_Temps_CAN = int32(zeros(1, 45));
      BMS_Cell_Voltages_CAN = int16(zeros(1, 100));
      GFDB_Isolation_State_CAN = uint8(0);
      MC_PS_Present_CAN = uint8(0);
      Batt_PS_Present_CAN = uint8(0);
      Cooling_Loop_Temps_CAN = int32(zeros(1, 5));
      MC_Cooling_FR_CAN = int16(0);
      Batt_Cooling_FR_CAN = int16(0);
      HIB_Comparison_Fault_CAN = false;
      HIB_ON_CAN = false;
      HUDL_ON_CAN = false;
      TMS_ON_CAN = false;
      GUB_ON_CAN = false;
      Acc_ON_CAN = false;
      Batt_12V_ON_CAN = false;
      Vicor_Input_Current_CAN = int16(0);
      LVSS_Temps_CAN = int32(zeros(1, 6));
      LVSS_Currents_CAN = int16(zeros(1, 6));
      Heartbeats_CAN = uint32([0, 0, 1, 1, 0]);
      Direction_Command1 = int16(0);
      Rolling_Counter1 = int16(0);
      Speed_Command1 = int16(0);
      Speed_Mode_Enable1 = int16(0);
      Torque_Limit_Command1 = int16(0);
      LS_Self_Test_In_A = false;
      LS_Self_Test_In_B = false;
      verify(BMS_Contactor_Command_uC_CAN == BMS_Contactor_Command.Open_Contactor);
    state Into_Key_Cycle
      BMS_Contactor_Closed_CAN = true;
      MC_ON = false;
    state MC_Incorrect
      GFDB_Isolation_State_CAN = 1;
    state Check
      verify(uC_State == UC_State.Super_Fault);
    (default) -> GFDB_Fault.Initialize
    GFDB_Fault.Initialize -> GFDB_Fault.Into_Key_Cycle : [
        | uC_State ~= UC_State.Preset
        | ]
    GFDB_Fault.Into_Key_Cycle -> GFDB_Fault.MC_Incorrect : [
        | uC_State ~= UC_State.Key_Cycle
        | ]
    GFDB_Fault.MC_Incorrect -> GFDB_Fault.Check : [
        | after(5, sec)
        | ]
  (default) -> Basic_Operation_Cycle [order 1] : [Active_Scenario_Index == 1]
  (default) -> Heartbeat_Fault [order 2] : [Active_Scenario_Index == 2]
  (default) -> MC_EN_Fault [order 3] : [Active_Scenario_Index == 3]
  (default) -> GFDB_Fault [order 4] : {assert(Active_Scenario_Index == 4,'The value of Scenario Parameter ''Active_Scenario_Index'' is not valid. Use the index of the scenario to specify it.')}
  data: LVSS_EN_uC input boolean size=[1]; Fault input boolean size=[1]; Super_Fault input boolean size=[1]; Watchdog input boolean size=[1]; uC_State input Enum: UC_State size=[1]; MC_EN_uC input boolean size=[1]; LED input boolean size=[1, 3]; LS_Self_Test_Out input boolean size=[1]; CAN_Self_Test input boolean size=[1]; MC_Self_Test input boolean size=[1]; Inverter_EN_uC_CAN input boolean size=[1]; Fault_to_MC_CAN input boolean size=[1]; Inverter_DC_uC_CAN input boolean size=[1]; Torque_Request_CAN input int16 size=[1]; BMS_Contactor_Command_uC_CAN input Enum: BMS_Contactor_Command size=[1]; MC_PS_Request_uC_CAN input uint8 size=[1]; Batt_PS_Request_uC_CAN input uint8 size=[1]; HIB_EN_uC_CAN input boolean size=[1]; HUDL_EN_uC_CAN input boolean size=[1]; TMS_EN_uC_CAN input boolean size=[1]; GUB_EN_uC_CAN input boolean size=[1]; Acc_EN_uC_CAN input boolean size=[1]; Batt_12V_EN_uC_CAN input boolean size=[1]; Direction_Command_uC_CAN input int16 size=[1]; Rolling_Counter_uC_CAN input int16 size=[1]; Speed_Command_uC_CAN input int16 size=[1]; Speed_Mode_Enable_uC_CAN input int16 size=[1]; Torque_Limit_Command_uC_CAN input int16 size=[1]; Ignition_LS_A output boolean size=[1]; Ignition_LS_B output boolean size=[1]; ESTOP_LS_A output boolean size=[1]; ESTOP_LS_B output boolean size=[1]; MC_ON output boolean size=[1]; Start_CAN output boolean size=[1]; Interlock output boolean size=[1]; LVSS_ON_CAN output boolean size=[1]; Brake_CAN output boolean size=[1]; Forward_EN_CAN output boolean size=[1]; MC_VSM_State_CAN output Enum: MC_VSM_State size=[1]; MC_DC_State_CAN output Enum: MC_DC_State size=[1]; Throttle_CAN output int16 size=[1]; BMS_Contactor_Closed_CAN output boolean size=[1]; BMS_Cell_Temps_CAN output int32 size=[1, 45]; BMS_Cell_Voltages_CAN output int16 size=[1, 100]; GFDB_Isolation_State_CAN output uint8 size=[1]; MC_PS_Present_CAN output uint8 size=[1]; Batt_PS_Present_CAN output uint8 size=[1]; Cooling_Loop_Temps_CAN output int32 size=[1, 5]; MC_Cooling_FR_CAN output int16 size=[1]; Batt_Cooling_FR_CAN output int16 size=[1]; HIB_Comparison_Fault_CAN output boolean size=[1]; HIB_ON_CAN output boolean size=[1]; HUDL_ON_CAN output boolean size=[1]; TMS_ON_CAN output boolean size=[1]; GUB_ON_CAN output boolean size=[1]; Acc_ON_CAN output boolean size=[1]; Batt_12V_ON_CAN output boolean size=[1]; Vicor_Input_Current_CAN output int16 size=[1]; LVSS_Temps_CAN output int32 size=[1, 6]; LVSS_Currents_CAN output int16 size=[1, 6]; Heartbeats_CAN output uint32 size=[1, 5]; Direction_Command1 output int16 size=[1]; Rolling_Counter1 output int16 size=[1]; Speed_Command1 output int16 size=[1]; Speed_Mode_Enable1 output int16 size=[1]; Torque_Limit_Command1 output int16 size=[1]; LS_Self_Test_In_A output boolean size=[1]; LS_Self_Test_In_B output boolean size=[1]; Active_Scenario_Index parameter =4
